simulink model "bu01_2018b"  (R2018b)
settings: Solver=VariableStepAuto  StartTime=0.0  StopTime=10.0  RelTol=1e-3
model workspace (MAT data in the model file):
  Ixx = 0.8
  Iyy = 2.075
  Izz = 1.25
  Mass = 11.5
libraries: aerolibutil x6, sharedtransform x4, simulink x3, sharedutil x3, shared6dof x1
(part 1 of 2)
settings Model: Creator=Administrator  LastModifiedBy=39926
settings DataIOCC: ReturnWorkspaceOutputs=on

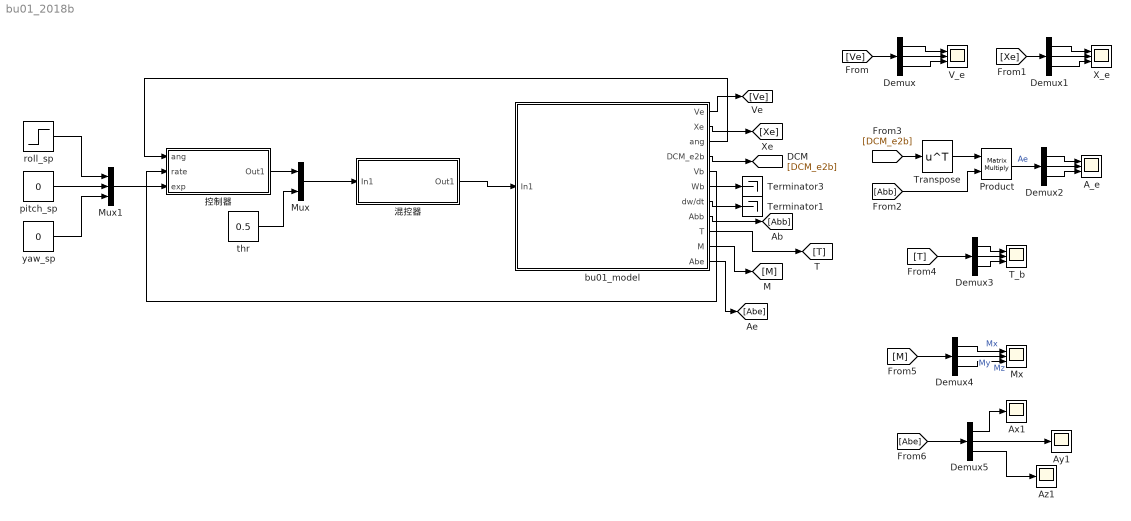
== system bu01_2018b ==
  A_e : Scope  NumInputPorts=3
  Ax1 : Scope
  Ay1 : Scope
  Az1 : Scope
  Demux{,1..5} (6 alike) : Demux  Outputs=3
  Mux : Mux  Inputs=2
  Mux1 : Mux  Inputs=3
  Mx : Scope  NumInputPorts=3
  Product : Product  Multiplication=Matrix(*)
  T_b : Scope  NumInputPorts=3
  Terminator1 : Terminator
  Terminator3 : Terminator
  Transpose : Math  Operator=transpose  SaturateOnIntegerOverflow=on
  V_e : Scope  NumInputPorts=3
  X_e : Scope  NumInputPorts=3
  bu01_model : Subsystem
  pitch_sp : Constant  Value=0
  roll_sp : Step  After=0  SampleTime=0
  thr : Constant  Value=0.5
  yaw_sp : Constant  Value=0
  控制器 : Subsystem
  混控器 : Subsystem
  wires:
  bu01_model/8(Abb) -> [Abb]
  bu01_model/7(dw/dt) -> Terminator1/1
  bu01_model/4(DCM_e2b) -> [DCM_e2b]
  bu01_model/5(Vb) -> Terminator3/1
  混控器/1(Out1) -> bu01_model/1(In1)
  Mux/1 -> 混控器/1(In1)
  bu01_model/3(ang) -> 控制器/1(ang)
  bu01_model/6(Wb) -> 控制器/2(rate)
  Mux1/1 -> 控制器/3(exp)
  控制器/1(Out1) -> Mux/1
  thr/1 -> Mux/2
  bu01_model/2(Xe) -> [Xe]
  Demux/1 -> V_e/1
  bu01_model/1(Ve) -> [Ve]
  [Ve] -> Demux/1
  [Xe] -> Demux1/1
  Demux1/1 -> X_e/1
  Demux1/2 -> X_e/2
  Demux1/3 -> X_e/3
  [DCM_e2b] -> Transpose/1
  Transpose/1 -> Product/1
  [Abb] -> Product/2
  Product/1 -> Demux2/1  "Ae"
  Demux2/1 -> A_e/1
  Demux2/2 -> A_e/2
  bu01_model/9(T) -> [T]
  bu01_model/10(M) -> [M]
  Demux3/3 -> T_b/3
  Demux3/2 -> T_b/2
  Demux3/1 -> T_b/1
  [T] -> Demux3/1
  [M] -> Demux4/1
  Demux4/1 -> Mx/1  "Mx"
  Demux4/2 -> Mx/2  "My"
  Demux4/3 -> Mx/3  "Mz"
  Demux2/3 -> A_e/3
  bu01_model/11(Abe) -> [Abe]
  Demux5/3 -> Az1/1
  Demux5/2 -> Ay1/1
  Demux5/1 -> Ax1/1
  [Abe] -> Demux5/1
  roll_sp/1 -> Mux1/1
  pitch_sp/1 -> Mux1/2
  yaw_sp/1 -> Mux1/3
  Demux/2 -> V_e/2
  Demux/3 -> V_e/3

== system bu01_2018b/bu01_model ==
  In1 : Inport
  6DOF (Quaternion) : shared6dof/6DOF (Euler Angles)  units=Metric (MKS)  mtype=Fixed  rep=Quaternion  xme_0=[0 0 0]  Vm_0=[0 0 0]  eul_0=[0 0 0]  pm_0=[0 0 0]  mass_0=Mass  mass_e=0.5  mass_f=2.0  inertia=[Ixx 0 0; 0 Iyy 0;0 0 Izz]  inertia_e=eye(3)  inertia_f=2*eye(3)  k_quat=1.0  vre_flag=on  abi_flag=on  aMode=0  xme_statename=''  Vm_statename=''  eul_statename=''  quat_statename=''  pm_statename=''  mass_statename=''
      settings: SourceProductBaseCode=AE
  力矩方程 : Subsystem
  推力方程 : Subsystem
  Ve : Outport
  Xe : Outport  Port=2
  ang : Outport  Port=3
  DCM_e2b : Outport  Port=4
  Vb : Outport  Port=5
  Wb : Outport  Port=6
  dw/dt : Outport  Port=7
  Abb : Outport  Port=8
  T : Outport  Port=9
  M : Outport  Port=10
  Abe : Outport  Port=11
  wires:
  力矩方程/1(Out1) -> M/1, 6DOF (Quaternion)/2
  6DOF (Quaternion)/1 -> Ve/1
  6DOF (Quaternion)/3 -> ang/1
  6DOF (Quaternion)/2 -> Xe/1
  6DOF (Quaternion)/4 -> 推力方程/2(DCM_e2b), DCM_e2b/1
  推力方程/1(Out1) -> T/1, 6DOF (Quaternion)/1
  6DOF (Quaternion)/7 -> dw/dt/1
  6DOF (Quaternion)/8 -> Abb/1
  6DOF (Quaternion)/5 -> Vb/1
  6DOF (Quaternion)/6 -> Wb/1
  In1/1 -> 推力方程/1(In1), 力矩方程/1(In1)
  6DOF (Quaternion)/9 -> Abe/1

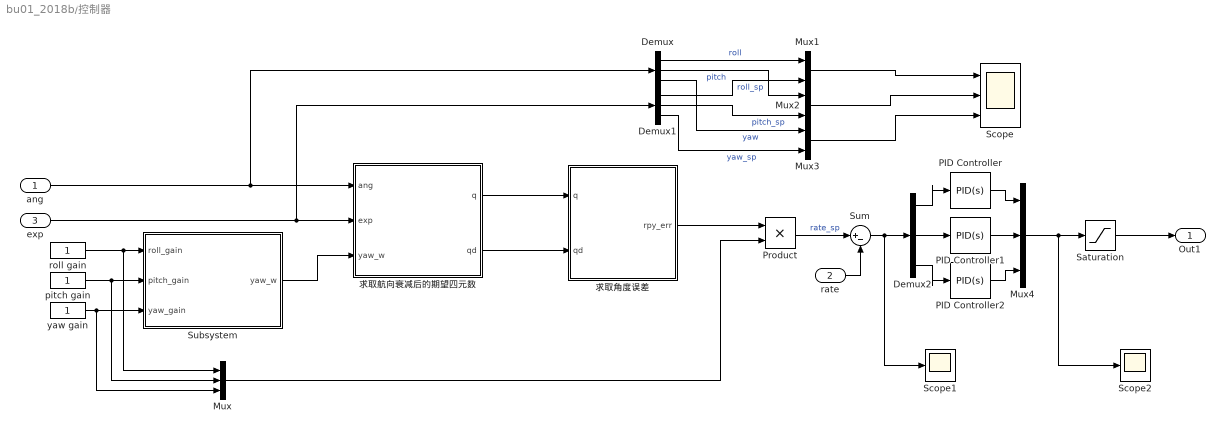
== system bu01_2018b/控制器 ==
  ang : Inport
  rate : Inport  Port=2
  exp : Inport  Port=3
  Demux : Demux  Outputs=3
  Demux1 : Demux  Outputs=3
  Demux2 : Demux  Outputs=3
  Mux : Mux  Inputs=3
  Mux1 : Mux  Inputs=2
  Mux2 : Mux  Inputs=2
  Mux3 : Mux  Inputs=2
  Mux4 : Mux  Inputs=3
  PID Controller : simulink/Continuous/PID Controller  Controller=PID  Form=Parallel  TimeDomain=Continuous-time  SampleTime=-1  IntegratorMethod=Forward Euler  FilterMethod=Forward Euler  ControllerParametersSource=internal  P=0.1  I=0.1  D=0  UseFilter=on  N=100  TunerSelectOption=Transfer Function Based (PID Tuner App)  InitialConditionSource=internal  InitialConditionForIntegrator=0  InitialConditionForFilter=0  DifferentiatorICPrevScaledInput=0  ExternalReset=none  TrackingMode=off  Kt=1  LimitOutput=off  UpperSaturationLimit=inf  LowerSaturationLimit=-inf  LinearizeAsGain=on  AntiWindupMode=none  Kb=1  POutMin=[]  POutMax=[]  IOutMin=[]  IOutMax=[]  DOutMin=[]  DOutMax=[]  NOutMin=[]  NOutMax=[]  SumOutMin=[]  SumOutMax=[]  SaturationOutMin=[]  SaturationOutMax=[]  PParamMin=[]  PParamMax=[]  IParamMin=[]  IParamMax=[]  DParamMin=[]  DParamMax=[]  NParamMin=[]  NParamMax=[]  KbParamMin=[]  KbParamMax=[]  KtParamMin=[]  KtParamMax=[]  KbOutMin=[]  KbOutMax=[]  KtOutMin=[]  KtOutMax=[]  IntegratorOutMin=[]  IntegratorOutMax=[]  FilterOutMin=[]  FilterOutMax=[]  SumI1OutMin=[]  SumI1OutMax=[]  SumI2OutMin=[]  SumI2OutMax=[]  SumI3OutMin=[]  SumI3OutMax=[]  SumI4OutMin=[]  SumI4OutMax=[]  SumDOutMin=[]  SumDOutMax=[]  DifferentiatorOutMin=[]  DifferentiatorOutMax=[]  FilterDiffOutCoefMin=[]  FilterDiffOutCoefMax=[]  ReciprocalOutMin=[]  ReciprocalOutMax=[]  SumDenOutMin=[]  SumDenOutMax=[]  SumNumOutMin=[]  SumNumOutMax=[]  DivideOutMin=[]  DivideOutMax=[]  IntegratorContinuousStateAttributes=''  IntegratorStateMustResolveToSignalObject=off  IntegratorRTWStateStorageClass=Auto  FilterContinuousStateAttributes=''  FilterStateMustResolveToSignalObject=off  FilterRTWStateStorageClass=Auto  ParallelPVariant=InternalParameters  IdealPVariant=Disabled  IVariant=InternalParameters  DVariant=InternalParameters  IntegratorVariant=Continuous  SatVariant=Disabled  AWVariant=Passthrough  PCopyVariant=Disabled  TRVariant=Disabled  FdbkBlocksVariant=Forward  IdealPFdbkVariant=Disabled  SatFdbkVariant=Disabled  DerivativeFilterVariant=ContFilter  NVariant=InternalParameters  NCopyVariant=Disabled  FilterICVariant=InternalICsFilter  IntegratorICVariant=InternalICs  ExternalResetVariant=Disabled  TRSumVariant=Passthrough  SumFdbkVariant=Disabled  SumVariant=Sum_PID
  PID Controller1 : simulink/Continuous/PID Controller  Controller=PID  Form=Parallel  TimeDomain=Continuous-time  SampleTime=-1  IntegratorMethod=Forward Euler  FilterMethod=Forward Euler  ControllerParametersSource=internal  P=0.15  I=0.1  D=0  UseFilter=on  N=100  TunerSelectOption=Transfer Function Based (PID Tuner App)  InitialConditionSource=internal  InitialConditionForIntegrator=0  InitialConditionForFilter=0  DifferentiatorICPrevScaledInput=0  ExternalReset=none  TrackingMode=off  Kt=1  LimitOutput=off  UpperSaturationLimit=inf  LowerSaturationLimit=-inf  LinearizeAsGain=on  AntiWindupMode=none  Kb=1  POutMin=[]  POutMax=[]  IOutMin=[]  IOutMax=[]  DOutMin=[]  DOutMax=[]  NOutMin=[]  NOutMax=[]  SumOutMin=[]  SumOutMax=[]  SaturationOutMin=[]  SaturationOutMax=[]  PParamMin=[]  PParamMax=[]  IParamMin=[]  IParamMax=[]  DParamMin=[]  DParamMax=[]  NParamMin=[]  NParamMax=[]  KbParamMin=[]  KbParamMax=[]  KtParamMin=[]  KtParamMax=[]  KbOutMin=[]  KbOutMax=[]  KtOutMin=[]  KtOutMax=[]  IntegratorOutMin=[]  IntegratorOutMax=[]  FilterOutMin=[]  FilterOutMax=[]  SumI1OutMin=[]  SumI1OutMax=[]  SumI2OutMin=[]  SumI2OutMax=[]  SumI3OutMin=[]  SumI3OutMax=[]  SumI4OutMin=[]  SumI4OutMax=[]  SumDOutMin=[]  SumDOutMax=[]  DifferentiatorOutMin=[]  DifferentiatorOutMax=[]  FilterDiffOutCoefMin=[]  FilterDiffOutCoefMax=[]  ReciprocalOutMin=[]  ReciprocalOutMax=[]  SumDenOutMin=[]  SumDenOutMax=[]  SumNumOutMin=[]  SumNumOutMax=[]  DivideOutMin=[]  DivideOutMax=[]  IntegratorContinuousStateAttributes=''  IntegratorStateMustResolveToSignalObject=off  IntegratorRTWStateStorageClass=Auto  FilterContinuousStateAttributes=''  FilterStateMustResolveToSignalObject=off  FilterRTWStateStorageClass=Auto  ParallelPVariant=InternalParameters  IdealPVariant=Disabled  IVariant=InternalParameters  DVariant=InternalParameters  IntegratorVariant=Continuous  SatVariant=Disabled  AWVariant=Passthrough  PCopyVariant=Disabled  TRVariant=Disabled  FdbkBlocksVariant=Forward  IdealPFdbkVariant=Disabled  SatFdbkVariant=Disabled  DerivativeFilterVariant=ContFilter  NVariant=InternalParameters  NCopyVariant=Disabled  FilterICVariant=InternalICsFilter  IntegratorICVariant=InternalICs  ExternalResetVariant=Disabled  TRSumVariant=Passthrough  SumFdbkVariant=Disabled  SumVariant=Sum_PID
  PID Controller2 : simulink/Continuous/PID Controller  Controller=PID  Form=Parallel  TimeDomain=Continuous-time  SampleTime=-1  IntegratorMethod=Forward Euler  FilterMethod=Forward Euler  ControllerParametersSource=internal  P=0.3  I=0.1  D=0  UseFilter=on  N=100  TunerSelectOption=Transfer Function Based (PID Tuner App)  InitialConditionSource=internal  InitialConditionForIntegrator=0  InitialConditionForFilter=0  DifferentiatorICPrevScaledInput=0  ExternalReset=none  TrackingMode=off  Kt=1  LimitOutput=off  UpperSaturationLimit=inf  LowerSaturationLimit=-inf  LinearizeAsGain=on  AntiWindupMode=none  Kb=1  POutMin=[]  POutMax=[]  IOutMin=[]  IOutMax=[]  DOutMin=[]  DOutMax=[]  NOutMin=[]  NOutMax=[]  SumOutMin=[]  SumOutMax=[]  SaturationOutMin=[]  SaturationOutMax=[]  PParamMin=[]  PParamMax=[]  IParamMin=[]  IParamMax=[]  DParamMin=[]  DParamMax=[]  NParamMin=[]  NParamMax=[]  KbParamMin=[]  KbParamMax=[]  KtParamMin=[]  KtParamMax=[]  KbOutMin=[]  KbOutMax=[]  KtOutMin=[]  KtOutMax=[]  IntegratorOutMin=[]  IntegratorOutMax=[]  FilterOutMin=[]  FilterOutMax=[]  SumI1OutMin=[]  SumI1OutMax=[]  SumI2OutMin=[]  SumI2OutMax=[]  SumI3OutMin=[]  SumI3OutMax=[]  SumI4OutMin=[]  SumI4OutMax=[]  SumDOutMin=[]  SumDOutMax=[]  DifferentiatorOutMin=[]  DifferentiatorOutMax=[]  FilterDiffOutCoefMin=[]  FilterDiffOutCoefMax=[]  ReciprocalOutMin=[]  ReciprocalOutMax=[]  SumDenOutMin=[]  SumDenOutMax=[]  SumNumOutMin=[]  SumNumOutMax=[]  DivideOutMin=[]  DivideOutMax=[]  IntegratorContinuousStateAttributes=''  IntegratorStateMustResolveToSignalObject=off  IntegratorRTWStateStorageClass=Auto  FilterContinuousStateAttributes=''  FilterStateMustResolveToSignalObject=off  FilterRTWStateStorageClass=Auto  ParallelPVariant=InternalParameters  IdealPVariant=Disabled  IVariant=InternalParameters  DVariant=InternalParameters  IntegratorVariant=Continuous  SatVariant=Disabled  AWVariant=Passthrough  PCopyVariant=Disabled  TRVariant=Disabled  FdbkBlocksVariant=Forward  IdealPFdbkVariant=Disabled  SatFdbkVariant=Disabled  DerivativeFilterVariant=ContFilter  NVariant=InternalParameters  NCopyVariant=Disabled  FilterICVariant=InternalICsFilter  IntegratorICVariant=InternalICs  ExternalResetVariant=Disabled  TRSumVariant=Passthrough  SumFdbkVariant=Disabled  SumVariant=Sum_PID
  Product : Product
  Saturation : Saturate  UpperLimit=1  LowerLimit=-1
  Scope : Scope  NumInputPorts=3
  Scope1 : Scope
  Scope2 : Scope
  Subsystem : Subsystem
  Sum : Sum  Inputs=|+-
  pitch gain : Constant
  roll gain : Constant
  yaw gain : Constant
  求取航向衰减后的期望四元数 : Subsystem
  求取角度误差 : Subsystem
  Out1 : Outport
  wires:
  ang/1 -> Demux/1, 求取航向衰减后的期望四元数/1(ang)
  exp/1 -> Demux1/1, 求取航向衰减后的期望四元数/2(exp)
  roll gain/1 -> Mux/1, Subsystem/1(roll_gain)
  pitch gain/1 -> Subsystem/2("pitch_gain "), Mux/2
  yaw gain/1 -> Subsystem/3(yaw_gain), Mux/3
  Subsystem/1(yaw_w) -> 求取航向衰减后的期望四元数/3("yaw_w ")
  求取航向衰减后的期望四元数/1(q) -> 求取角度误差/1(q)
  求取航向衰减后的期望四元数/2(qd) -> 求取角度误差/2(qd)
  求取角度误差/1(rpy_err) -> Product/1
  Mux/1 -> Product/2
  Product/1 -> Sum/1  "rate_sp"
  rate/1 -> Sum/2
  Sum/1 -> Scope1/1, Demux2/1
  Mux4/1 -> Scope2/1, Saturation/1
  Saturation/1 -> Out1/1
  Demux/1 -> Mux1/1  "roll"
  Demux1/1 -> Mux1/2  "roll_sp"
  Demux/2 -> Mux2/1  "pitch"
  Demux1/2 -> Mux2/2  "pitch_sp"
  Demux/3 -> Mux3/1  "yaw"
  Demux1/3 -> Mux3/2  "yaw_sp"
  Mux1/1 -> Scope/1
  Mux2/1 -> Scope/2
  Mux3/1 -> Scope/3
  Demux2/1 -> PID Controller/1
  Demux2/2 -> PID Controller1/1
  Demux2/3 -> PID Controller2/1
  PID Controller/1 -> Mux4/1
  PID Controller1/1 -> Mux4/2
  PID Controller2/1 -> Mux4/3

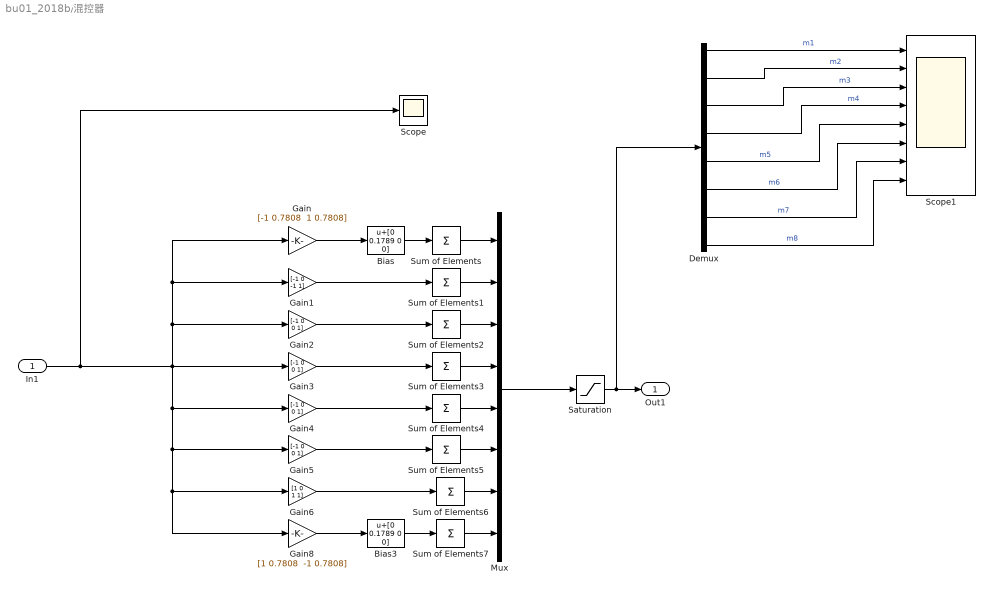
== system bu01_2018b/混控器 ==
  In1 : Inport
  Bias : Bias  Bias=[0 0.1789 0 0]
  Bias3 : Bias  Bias=[0 0.1789 0 0]
  Demux : Demux  Outputs=8
  Gain : Gain  Gain="[-1 0.7808  1 0.7808]"
  Gain1 : Gain  Gain="[-1 0  -1 1]"
  Gain{2..5} (4 alike) : Gain  Gain=[-1 0 0 1]
  Gain6 : Gain  Gain="[1 0  1 1]"
  Gain8 : Gain  Gain="[1 0.7808  -1 0.7808]"
  Mux : Mux  Inputs=8
  Saturation : Saturate  UpperLimit=1  LowerLimit=0
  Scope : Scope
  Scope1 : Scope  NumInputPorts=8
  Sum of Elements{,1..7} (8 alike) : Sum  Inputs=+
  Out1 : Outport
  wires:
  Sum of Elements/1 -> Mux/1
  Bias/1 -> Sum of Elements/1
  Gain2/1 -> Sum of Elements2/1
  Gain3/1 -> Sum of Elements3/1
  Gain5/1 -> Sum of Elements5/1
  Gain4/1 -> Sum of Elements4/1
  Mux/1 -> Saturation/1
  Gain/1 -> Bias/1
  Gain1/1 -> Sum of Elements1/1
  Gain6/1 -> Sum of Elements6/1
  Gain8/1 -> Bias3/1
  Bias3/1 -> Sum of Elements7/1
  Saturation/1 -> Demux/1, Out1/1
  Sum of Elements1/1 -> Mux/2
  Sum of Elements2/1 -> Mux/3
  Sum of Elements3/1 -> Mux/4
  Sum of Elements4/1 -> Mux/5
  Sum of Elements5/1 -> Mux/6
  Sum of Elements6/1 -> Mux/7
  Sum of Elements7/1 -> Mux/8
  In1/1 -> Scope/1, Gain3/1, Gain4/1, Gain5/1, Gain8/1, Gain6/1, Gain1/1, Gain/1, Gain2/1
  Demux/1 -> Scope1/1  "m1"
  Demux/2 -> Scope1/2  "m2"
  Demux/3 -> Scope1/3  "m3"
  Demux/4 -> Scope1/4  "m4"
  Demux/5 -> Scope1/5  "m5"
  Demux/6 -> Scope1/6  "m6"
  Demux/7 -> Scope1/7  "m7"
  Demux/8 -> Scope1/8  "m8"

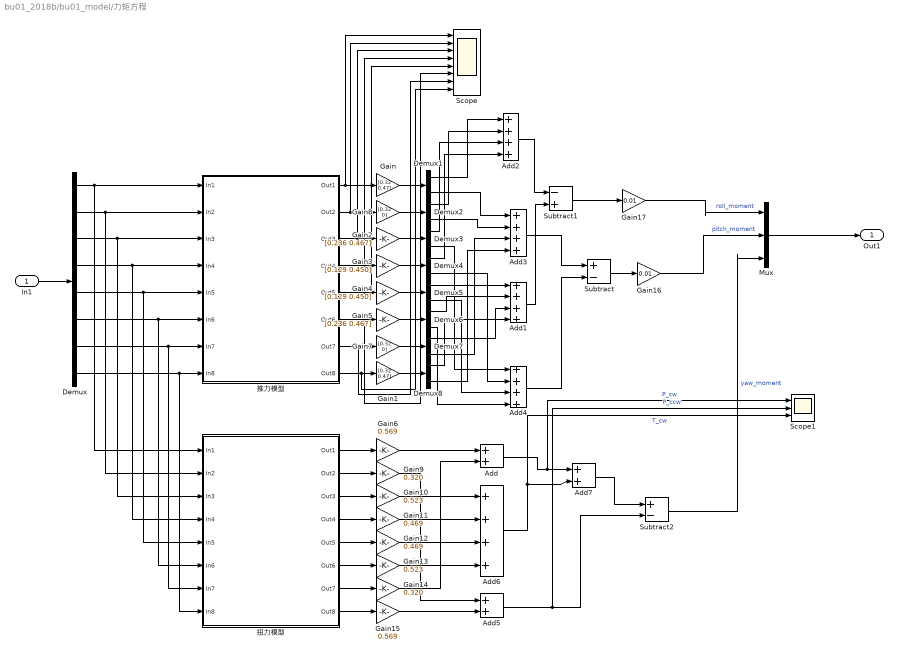
== system bu01_2018b/bu01_model/力矩方程 ==
  In1 : Inport
  Add : Sum
  Add{1..4} (4 alike) : Sum  Inputs=4
  Add5 : Sum
  Add6 : Sum  Inputs=++++
  Add7 : Sum
  Demux : Demux  Outputs=8
  Demux{1..8} (8 alike) : Demux  Outputs=2
  Gain : Gain  Gain=[0.32 0.47]
  Gain1 : Gain  Gain=[0.32 0.47]
  Gain10 : Gain  Gain=0.523
  Gain11 : Gain  Gain=0.469
  Gain12 : Gain  Gain=0.469
  Gain13 : Gain  Gain=0.523
  Gain14 : Gain  Gain=0.320
  Gain15 : Gain  Gain=0.569
  Gain16 : Gain  Gain=0.01
  Gain17 : Gain  Gain=0.01
  Gain2 : Gain  Gain=[0.236 0.467]
  Gain3 : Gain  Gain=[0.129 0.450]
  Gain4 : Gain  Gain=[0.129 0.450]
  Gain5 : Gain  Gain=[0.236 0.467]
  Gain6 : Gain  Gain=0.569
  Gain7 : Gain  Gain=[0.32 0]
  Gain8 : Gain  Gain=[0.32 0]
  Gain9 : Gain  Gain=0.320
  Mux : Mux  Inputs=3
  Scope : Scope  NumInputPorts=8
  Scope1 : Scope  NumInputPorts=3
  Subtract : Sum  Inputs=+-
  Subtract1 : Sum  Inputs=-+
  Subtract2 : Sum  Inputs=+-
  扭力模型 : Subsystem
  推力模型 : Subsystem
  Out1 : Outport
  wires:
  In1/1 -> Demux/1
  Demux/1 -> 推力模型/1(In1), 扭力模型/1(In1)
  Demux/2 -> 扭力模型/2(In2), 推力模型/2(In2)
  Demux/3 -> 推力模型/3(In3), 扭力模型/3(In3)
  Demux/4 -> 推力模型/4(In4), 扭力模型/4(In4)
  Demux/5 -> 推力模型/5(In5), 扭力模型/5(In5)
  Demux/6 -> 扭力模型/6(In6), 推力模型/6(In6)
  Demux/7 -> 扭力模型/7(In7), 推力模型/7(In7)
  Demux/8 -> 扭力模型/8(In8), 推力模型/8(In8)
  推力模型/1(Out1) -> Scope/1, Gain/1
  推力模型/8(Out8) -> Scope/8, Gain1/1
  推力模型/4(Out4) -> Scope/4, Gain3/1
  推力模型/5(Out5) -> Scope/5, Gain4/1
  推力模型/6(Out6) -> Scope/6, Gain5/1
  推力模型/7(Out7) -> Scope/7, Gain7/1
  Gain/1 -> Demux1/1
  Gain8/1 -> Demux2/1
  Gain2/1 -> Demux3/1
  Gain3/1 -> Demux4/1
  Gain4/1 -> Demux5/1
  Gain5/1 -> Demux6/1
  Gain7/1 -> Demux7/1
  Gain1/1 -> Demux8/1
  Demux1/1 -> Add2/1
  Demux2/1 -> Add2/2
  Demux3/1 -> Add2/3
  Demux4/1 -> Add2/4
  Demux5/1 -> Add1/1
  Demux6/1 -> Add1/2
  Demux7/1 -> Add1/3
  Demux8/1 -> Add1/4
  Add2/1 -> Subtract1/1
  Add1/1 -> Subtract1/2
  Demux1/2 -> Add3/1
  Demux2/2 -> Add3/2
  Demux7/2 -> Add3/3
  Demux8/2 -> Add3/4
  Demux3/2 -> Add4/1
  Demux4/2 -> Add4/2
  Demux5/2 -> Add4/3
  Demux6/2 -> Add4/4
  Add3/1 -> Subtract/1
  Add4/1 -> Subtract/2
  扭力模型/1(Out1) -> Gain6/1
  扭力模型/2(Out2) -> Gain9/1
  扭力模型/3(Out3) -> Gain10/1
  扭力模型/4(Out4) -> Gain11/1
  扭力模型/5(Out5) -> Gain12/1
  扭力模型/6(Out6) -> Gain13/1
  扭力模型/7(Out7) -> Gain14/1
  扭力模型/8(Out8) -> Gain15/1
  Gain6/1 -> Add/1
  Gain14/1 -> Add/2
  Gain15/1 -> Add5/2
  Gain9/1 -> Add5/1
  Gain13/1 -> Add6/4
  Gain12/1 -> Add6/3
  Gain11/1 -> Add6/2
  Gain10/1 -> Add6/1
  Add/1 -> Scope1/1, Add7/1  "P_cw"
  Add7/1 -> Subtract2/1
  Add5/1 -> Scope1/2, Subtract2/2  "P_ccw"
  Subtract2/1 -> Mux/3  "yaw_moment"
  Mux/1 -> Out1/1
  Subtract/1 -> Gain16/1
  Gain16/1 -> Mux/2  "pitch_moment"
  Subtract1/1 -> Gain17/1
  Gain17/1 -> Mux/1  "roll_moment"
  推力模型/2(Out2) -> Gain8/1, Scope/2
  推力模型/3(Out3) -> Scope/3, Gain2/1
  Add6/1 -> Scope1/3, Add7/2  "T_cw"

== system bu01_2018b/bu01_model/推力方程 ==
  In1 : Inport
  DCM_e2b : Inport  Port=2
  Add : Sum  Inputs=8
  Add1 : Sum
  Constant : Constant  Value=0
  Constant1 : Constant  Value=0
  Demux : Demux  Outputs=8
  Gain : Gain  Gain=-0.01
  Mux : Mux  Inputs=3
  Product : Product  Multiplication=Matrix(*)
  aircraft_mg : Constant  Value=[0 0 115.7]
  动力模型 : Subsystem
  Out1 : Outport
  wires:
  In1/1 -> Demux/1
  Demux/1 -> 动力模型/1(In1)
  Demux/2 -> 动力模型/2(In2)
  Demux/3 -> 动力模型/3(In3)
  Demux/4 -> 动力模型/4(In4)
  Demux/5 -> 动力模型/5(In5)
  Demux/6 -> 动力模型/6(In6)
  Demux/7 -> 动力模型/7(In7)
  Demux/8 -> 动力模型/8(In8)
  动力模型/1(Out1) -> Add/1
  动力模型/2(Out2) -> Add/2
  动力模型/3(Out3) -> Add/3
  动力模型/4(Out4) -> Add/4
  动力模型/5(Out5) -> Add/5
  动力模型/7(Out7) -> Add/7
  动力模型/6(Out6) -> Add/6
  动力模型/8(Out8) -> Add/8
  Constant/1 -> Mux/1
  Constant1/1 -> Mux/2
  Add/1 -> Gain/1
  Gain/1 -> Mux/3
  DCM_e2b/1 -> Product/1
  aircraft_mg/1 -> Product/2
  Product/1 -> Add1/2
  Mux/1 -> Add1/1
  Add1/1 -> Out1/1

== system bu01_2018b/控制器/Subsystem ==
  note: 将比例增益当做系统时间常数，用其比例关系作为控制器衰减比例
  roll_gain : Inport
  "pitch_gain " : Inport  Port=2
  yaw_gain : Inport  Port=3
  Add : Sum
  Divide : Product  Inputs=*/
  Gain : Gain  Gain=0.5
  Saturation : Saturate  UpperLimit=1  LowerLimit=0
  yaw_w : Outport
  wires:
  roll_gain/1 -> Add/1
  Add/1 -> Gain/1
  "pitch_gain "/1 -> Add/2
  Gain/1 -> Divide/2
  yaw_gain/1 -> Divide/1
  Divide/1 -> Saturation/1
  Saturation/1 -> yaw_w/1

== system bu01_2018b/控制器/求取航向衰减后的期望四元数 ==
  ang : Inport
  exp : Inport  Port=2
  "yaw_w " : Inport  Port=3
  MATLAB Function : MATLAB Function  TreatAsAtomicUnit=on
  Quaternion Normalize : sharedutil/Quaternion Normalize  aMode=aMode
      settings: SourceProductName=Aerospace Blockset  SourceProductBaseCode=AE
  求取只要倾斜的运动的期望四元数 : Subsystem
  求取绕机体Z轴旋转的误差四元数 : Subsystem
  获取地球系下当前机体系Z轴矢量 : Subsystem
  获取地球系下期望机体系Z轴矢量 : Subsystem
  计算航向衰减后的期望四元数 : Subsystem
  q : Outport
  qd : Outport  Port=2
  wires:
  获取地球系下当前机体系Z轴矢量/2(e_z) -> MATLAB Function/1(src)
  ang/1 -> 获取地球系下当前机体系Z轴矢量/1(ang)
  exp/1 -> 获取地球系下期望机体系Z轴矢量/1(exp)
  获取地球系下当前机体系Z轴矢量/1(q) -> q/1, 求取只要倾斜的运动的期望四元数/1(q)
  获取地球系下期望机体系Z轴矢量/1(e_z_d) -> MATLAB Function/2(dst)
  获取地球系下期望机体系Z轴矢量/2("qd ") -> 求取绕机体Z轴旋转的误差四元数/2(qd), 求取只要倾斜的运动的期望四元数/3(qd)
  "yaw_w "/1 -> 计算航向衰减后的期望四元数/1(yaw_w)
  求取绕机体Z轴旋转的误差四元数/1(q_mix_sign) -> 计算航向衰减后的期望四元数/3(q_mix_sign)
  计算航向衰减后的期望四元数/1(qd) -> qd/1
  求取只要倾斜的运动的期望四元数/1(qd_red_update) -> 计算航向衰减后的期望四元数/2(q_red_update), 求取绕机体Z轴旋转的误差四元数/1(qd_red_update)
  MATLAB Function/1(q) -> Quaternion Normalize/1  "qd_red"
  Quaternion Normalize/1 -> 求取只要倾斜的运动的期望四元数/2(qd_red)

== system bu01_2018b/控制器/求取角度误差 ==
  q : Inport
  qd : Inport  Port=2
  Constant : Constant  Value=0
  Gain : Gain  Gain=-1
  Gain1 : Gain  Gain=2
  GreaterThanOrEqual : RelationalOperator  OutDataTypeStr=boolean  RndMeth=Simplest
  Quaternion Inverse : aerolibutil/Quaternion Inverse
      settings: SourceProductName=Aerospace Blockset
  Quaternion Multiplication : aerolibutil/Quaternion Multiplication
  Selector : Selector  InputPortWidth=4  IndexOptions=Index vector (dialog)  Indices=1  OutputSizes=1
  Selector1 : Selector  InputPortWidth=4  IndexOptions=Index vector (dialog)  Indices=[2 3 4]  OutputSizes=1
  Switch : Switch  Criteria=u2 > Threshold
  rpy_err : Outport
  wires:
  Quaternion Inverse/1 -> Quaternion Multiplication/1
  q/1 -> Quaternion Inverse/1
  Quaternion Multiplication/1 -> Selector1/1, Selector/1  "quat_err"
  qd/1 -> Quaternion Multiplication/2
  Selector/1 -> GreaterThanOrEqual/1
  Constant/1 -> GreaterThanOrEqual/2
  GreaterThanOrEqual/1 -> Switch/2
  Selector1/1 -> Switch/1, Gain/1
  Gain/1 -> Switch/3
  Switch/1 -> Gain1/1
  Gain1/1 -> rpy_err/1  "ang_err"

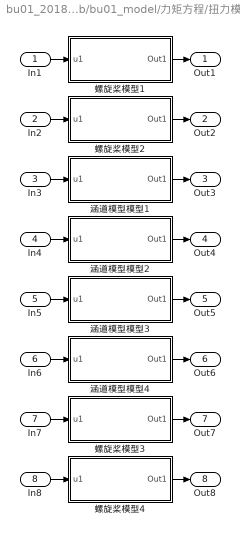
== system bu01_2018b/bu01_model/力矩方程/扭力模型 ==
  In1 : Inport
  In2 : Inport  Port=2
  In3 : Inport  Port=3
  In4 : Inport  Port=4
  In5 : Inport  Port=5
  In6 : Inport  Port=6
  In7 : Inport  Port=7
  In8 : Inport  Port=8
  涵道模型模型1 : Subsystem
  涵道模型模型2 : Subsystem
  涵道模型模型3 : Subsystem
  涵道模型模型4 : Subsystem
  螺旋桨模型1 : Subsystem
  螺旋桨模型2 : Subsystem
  螺旋桨模型3 : Subsystem
  螺旋桨模型4 : Subsystem
  Out1 : Outport
  Out2 : Outport  Port=2
  Out3 : Outport  Port=3
  Out4 : Outport  Port=4
  Out5 : Outport  Port=5
  Out6 : Outport  Port=6
  Out7 : Outport  Port=7
  Out8 : Outport  Port=8
  wires:
  In3/1 -> 涵道模型模型1/1(u1)
  涵道模型模型2/1(Out1) -> Out4/1
  涵道模型模型3/1(Out1) -> Out5/1
  螺旋桨模型1/1(Out1) -> Out1/1
  In7/1 -> 螺旋桨模型3/1(u1)
  涵道模型模型1/1(Out1) -> Out3/1
  In4/1 -> 涵道模型模型2/1(u1)
  In5/1 -> 涵道模型模型3/1(u1)
  螺旋桨模型3/1(Out1) -> Out7/1
  In2/1 -> 螺旋桨模型2/1(u1)
  螺旋桨模型2/1(Out1) -> Out2/1
  In6/1 -> 涵道模型模型4/1(u1)
  涵道模型模型4/1(Out1) -> Out6/1
  螺旋桨模型4/1(Out1) -> Out8/1
  In8/1 -> 螺旋桨模型4/1(u1)
  In1/1 -> 螺旋桨模型1/1(u1)

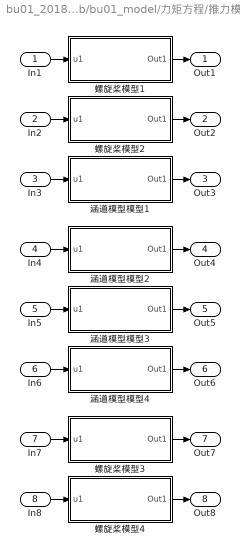
== system bu01_2018b/bu01_model/力矩方程/推力模型 ==
  In1 : Inport
  In2 : Inport  Port=2
  In3 : Inport  Port=3
  In4 : Inport  Port=4
  In5 : Inport  Port=5
  In6 : Inport  Port=6
  In7 : Inport  Port=7
  In8 : Inport  Port=8
  涵道模型模型1 : Subsystem
  涵道模型模型2 : Subsystem
  涵道模型模型3 : Subsystem
  涵道模型模型4 : Subsystem
  螺旋桨模型1 : Subsystem
  螺旋桨模型2 : Subsystem
  螺旋桨模型3 : Subsystem
  螺旋桨模型4 : Subsystem
  Out1 : Outport
  Out2 : Outport  Port=2
  Out3 : Outport  Port=3
  Out4 : Outport  Port=4
  Out5 : Outport  Port=5
  Out6 : Outport  Port=6
  Out7 : Outport  Port=7
  Out8 : Outport  Port=8
  wires:
  In2/1 -> 螺旋桨模型2/1(u1)
  In3/1 -> 涵道模型模型1/1(u1)
  In7/1 -> 螺旋桨模型3/1(u1)
  In1/1 -> 螺旋桨模型1/1(u1)
  螺旋桨模型1/1(Out1) -> Out1/1
  涵道模型模型1/1(Out1) -> Out3/1
  In8/1 -> 螺旋桨模型4/1(u1)
  涵道模型模型3/1(Out1) -> Out5/1
  螺旋桨模型4/1(Out1) -> Out8/1
  In6/1 -> 涵道模型模型4/1(u1)
  螺旋桨模型3/1(Out1) -> Out7/1
  螺旋桨模型2/1(Out1) -> Out2/1
  In5/1 -> 涵道模型模型3/1(u1)
  涵道模型模型4/1(Out1) -> Out6/1
  涵道模型模型2/1(Out1) -> Out4/1
  In4/1 -> 涵道模型模型2/1(u1)

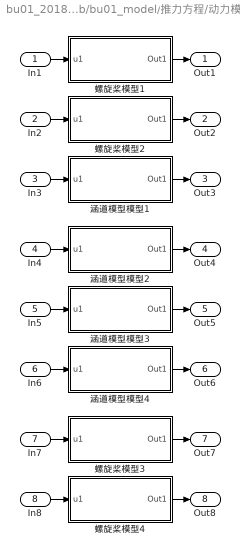
== system bu01_2018b/bu01_model/推力方程/动力模型 ==
  In1 : Inport
  In2 : Inport  Port=2
  In3 : Inport  Port=3
  In4 : Inport  Port=4
  In5 : Inport  Port=5
  In6 : Inport  Port=6
  In7 : Inport  Port=7
  In8 : Inport  Port=8
  涵道模型模型1 : Subsystem
  涵道模型模型2 : Subsystem
  涵道模型模型3 : Subsystem
  涵道模型模型4 : Subsystem
  螺旋桨模型1 : Subsystem
  螺旋桨模型2 : Subsystem
  螺旋桨模型3 : Subsystem
  螺旋桨模型4 : Subsystem
  Out1 : Outport
  Out2 : Outport  Port=2
  Out3 : Outport  Port=3
  Out4 : Outport  Port=4
  Out5 : Outport  Port=5
  Out6 : Outport  Port=6
  Out7 : Outport  Port=7
  Out8 : Outport  Port=8
  wires:
  In2/1 -> 螺旋桨模型2/1(u1)
  In3/1 -> 涵道模型模型1/1(u1)
  In7/1 -> 螺旋桨模型3/1(u1)
  In1/1 -> 螺旋桨模型1/1(u1)
  螺旋桨模型1/1(Out1) -> Out1/1
  涵道模型模型1/1(Out1) -> Out3/1
  In8/1 -> 螺旋桨模型4/1(u1)
  涵道模型模型3/1(Out1) -> Out5/1
  螺旋桨模型4/1(Out1) -> Out8/1
  In6/1 -> 涵道模型模型4/1(u1)
  螺旋桨模型3/1(Out1) -> Out7/1
  螺旋桨模型2/1(Out1) -> Out2/1
  In5/1 -> 涵道模型模型3/1(u1)
  涵道模型模型4/1(Out1) -> Out6/1
  涵道模型模型2/1(Out1) -> Out4/1
  In4/1 -> 涵道模型模型2/1(u1)

== system bu01_2018b/控制器/求取航向衰减后的期望四元数/求取只要倾斜的运动的期望四元数 ==
  note: 没有航向旋转的情况
  q : Inport
  qd_red : Inport  Port=2
  qd : Inport  Port=3
  Constant : Constant  Value=1-1e-5
  Demux : Demux  Outputs=2
  GreaterThan : RelationalOperator  Operator=>  OutDataTypeStr=boolean  RndMeth=Simplest
  GreaterThan1 : RelationalOperator  Operator=>  OutDataTypeStr=boolean  RndMeth=Simplest
  OR : Logic  Operator=OR  IconShape=distinctive  AllPortsSameDT=off  OutDataTypeStr=boolean
  Quaternion Multiplication : aerolibutil/Quaternion Multiplication
  Selector : Selector  InputPortWidth=4  IndexOptions=Index vector (dialog)  Indices=[2 3]  OutputSizes=1
  Switch : Switch  Criteria=u2 > Threshold
  qd_red_update : Outport
  wires:
  qd/1 -> Switch/1
  Constant/1 -> GreaterThan/2, GreaterThan1/2
  GreaterThan/1 -> OR/1
  q/1 -> Quaternion Multiplication/2
  GreaterThan1/1 -> OR/2
  qd_red/1 -> Quaternion Multiplication/1, Selector/1
  OR/1 -> Switch/2
  Demux/2 -> GreaterThan1/1
  Demux/1 -> GreaterThan/1
  Selector/1 -> Demux/1
  Quaternion Multiplication/1 -> Switch/3
  Switch/1 -> qd_red_update/1  "qd_red_update"

== system bu01_2018b/控制器/求取航向衰减后的期望四元数/求取绕机体Z轴旋转的误差四元数 ==
  qd_red_update : Inport
  qd : Inport  Port=2
  Constant1 : Constant  Value=0
  Gain : Gain  Gain=-1
  GreaterThan2 : RelationalOperator  OutDataTypeStr=boolean  RndMeth=Simplest
  Quaternion Inverse : aerolibutil/Quaternion Inverse
      settings: SourceProductName=Aerospace Blockset
  Quaternion Multiplication1 : aerolibutil/Quaternion Multiplication
  Selector1 : Selector  InputPortWidth=4  IndexOptions=Index vector (dialog)  Indices=1  OutputSizes=1
  Switch1 : Switch  Criteria=u2 > Threshold
  q_mix_sign : Outport
  wires:
  qd/1 -> Quaternion Multiplication1/2
  Quaternion Multiplication1/1 -> Gain/1, Switch1/1, Selector1/1  "q_mix"
  Gain/1 -> Switch1/3
  Selector1/1 -> GreaterThan2/1
  GreaterThan2/1 -> Switch1/2
  Constant1/1 -> GreaterThan2/2
  Quaternion Inverse/1 -> Quaternion Multiplication1/1
  qd_red_update/1 -> Quaternion Inverse/1
  Switch1/1 -> q_mix_sign/1  "q_mix_sign"

== system bu01_2018b/控制器/求取航向衰减后的期望四元数/获取地球系下当前机体系Z轴矢量 ==
  ang : Inport
  Quaternion Normalize1 : sharedutil/Quaternion Normalize  aMode=aMode
      settings: SourceProductName=Aerospace Blockset  SourceProductBaseCode=AE
  Quaternions to Direction Cosine Matrix1 : sharedtransform/Quaternions to  Direction Cosine Matrix  aMode=aMode
      settings: SourceProductName=Aerospace Blockset  SourceProductBaseCode=AE
  Rotation Angles to Quaternions : sharedtransform/Rotation Angles to Quaternions  rotationOrder=XYZ  aMode=aMode
      settings: SourceProductName=Aerospace Blockset  SourceProductBaseCode=AE
  提取机体系Z轴在 导航系下的矢量1 : Selector  NumberOfDimensions=2  InputPortWidth=3  IndexOptions=Index vector (dialog),Index vector (dialog)  Indices=3,[1 2 3]  OutputSizes=1,1
  q : Outport
  e_z : Outport  Port=2
  wires:
  Quaternions to Direction Cosine Matrix1/1 -> 提取机体系Z轴在 导航系下的矢量1/1
  Quaternion Normalize1/1 -> q/1, Quaternions to Direction Cosine Matrix1/1
  Rotation Angles to Quaternions/1 -> Quaternion Normalize1/1
  ang/1 -> Rotation Angles to Quaternions/1
  提取机体系Z轴在 导航系下的矢量1/1 -> e_z/1

== system bu01_2018b/控制器/求取航向衰减后的期望四元数/获取地球系下期望机体系Z轴矢量 ==
  exp : Inport
  Quaternion Normalize : sharedutil/Quaternion Normalize  aMode=aMode
      settings: SourceProductName=Aerospace Blockset  SourceProductBaseCode=AE
  Quaternions to Direction Cosine Matrix : sharedtransform/Quaternions to  Direction Cosine Matrix  aMode=aMode
      settings: SourceProductName=Aerospace Blockset  SourceProductBaseCode=AE
  Rotation Angles to Quaternions1 : sharedtransform/Rotation Angles to Quaternions  rotationOrder=XYZ  aMode=aMode
      settings: SourceProductName=Aerospace Blockset  SourceProductBaseCode=AE
  提取机体系Z轴在 导航系下的矢量 : Selector  NumberOfDimensions=2  InputPortWidth=3  IndexOptions=Index vector (dialog),Index vector (dialog)  Indices=3,[1 2 3]  OutputSizes=1,1
  e_z_d : Outport
  "qd " : Outport  Port=2
  wires:
  Rotation Angles to Quaternions1/1 -> Quaternion Normalize/1
  Quaternion Normalize/1 -> "qd "/1, Quaternions to Direction Cosine Matrix/1
  Quaternions to Direction Cosine Matrix/1 -> 提取机体系Z轴在 导航系下的矢量/1
  提取机体系Z轴在 导航系下的矢量/1 -> e_z_d/1
  exp/1 -> Rotation Angles to Quaternions1/1

== system bu01_2018b/控制器/求取航向衰减后的期望四元数/计算航向衰减后的期望四元数 ==
  yaw_w : Inport
  q_red_update : Inport  Port=2
  q_mix_sign : Inport  Port=3
  Acos : Trigonometry  Operator=acos
  Acos1 : Trigonometry  Operator=asin
  Constant3 : Constant  Value=0
  Cos : Trigonometry  Operator=cos
  Cos1 : Trigonometry
  Demux1 : Demux  Outputs=2
  Mux : Mux
  Product : Product
  Product1 : Product
  Quaternion Multiplication2 : aerolibutil/Quaternion Multiplication
  Saturation : Saturate  UpperLimit=1  LowerLimit=-1
  Selector2 : Selector  InputPortWidth=4  IndexOptions=Index vector (dialog)  Indices=[1 4]  OutputSizes=1
  qd : Outport
  wires:
  Product/1 -> Cos/1
  Cos/1 -> Mux/1
  Cos1/1 -> Mux/4
  Saturation/1 -> Demux1/1
  yaw_w/1 -> Product1/2, Product/1
  Acos/1 -> Product/2
  Demux1/1 -> Acos/1
  Product1/1 -> Cos1/1
  Mux/1 -> Quaternion Multiplication2/2
  Quaternion Multiplication2/1 -> qd/1  "qd"
  Constant3/1 -> Mux/3, Mux/2
  Acos1/1 -> Product1/1
  q_red_update/1 -> Quaternion Multiplication2/1
  Demux1/2 -> Acos1/1
  Selector2/1 -> Saturation/1
  q_mix_sign/1 -> Selector2/1

== system bu01_2018b/bu01_model/力矩方程/扭力模型/涵道模型模型1 ==
  u1 : Inport
  Add : Sum
  Constant : Constant  Value=0
  Constant1 : Constant  Value=0.1023
  Constant2 : Constant  Value=0.1023
  Constant3 : Constant
  Gain : Gain  Gain=0.003
  Gain1 : Gain  Gain=0.09767
  Gain2 : Gain  Gain=20
  MATLAB Function : MATLAB Function  TreatAsAtomicUnit=on
  MATLAB Function1 : MATLAB Function  TreatAsAtomicUnit=on
  Out1 : Outport
  wires:
  MATLAB Function1/1(y) -> Gain1/1
  Constant2/1 -> MATLAB Function1/2(a)
  Constant3/1 -> MATLAB Function1/3(b)
  Constant1/1 -> MATLAB Function/3(b)
  Gain1/1 -> Add/2
  Constant/1 -> MATLAB Function/2(a)
  u1/1 -> MATLAB Function1/1(u), MATLAB Function/1(u)
  Gain/1 -> Add/1
  MATLAB Function/1(y) -> Gain/1
  Add/1 -> Gain2/1
  Gain2/1 -> Out1/1

== system bu01_2018b/bu01_model/力矩方程/扭力模型/涵道模型模型2 ==
  u1 : Inport
  Add : Sum
  Constant : Constant  Value=0
  Constant1 : Constant  Value=0.1023
  Constant2 : Constant  Value=0.1023
  Constant3 : Constant
  Gain : Gain  Gain=0.003
  Gain1 : Gain  Gain=0.09767
  Gain2 : Gain  Gain=20
  MATLAB Function : MATLAB Function  TreatAsAtomicUnit=on
  MATLAB Function1 : MATLAB Function  TreatAsAtomicUnit=on
  Out1 : Outport
  wires:
  Gain2/1 -> Out1/1
  Add/1 -> Gain2/1
  MATLAB Function/1(y) -> Gain/1
  Gain/1 -> Add/1
  u1/1 -> MATLAB Function/1(u), MATLAB Function1/1(u)
  Constant/1 -> MATLAB Function/2(a)
  Gain1/1 -> Add/2
  Constant1/1 -> MATLAB Function/3(b)
  Constant3/1 -> MATLAB Function1/3(b)
  Constant2/1 -> MATLAB Function1/2(a)
  MATLAB Function1/1(y) -> Gain1/1

== system bu01_2018b/bu01_model/力矩方程/扭力模型/涵道模型模型3 ==
  u1 : Inport
  Add : Sum
  Constant : Constant  Value=0
  Constant1 : Constant  Value=0.1023
  Constant2 : Constant  Value=0.1023
  Constant3 : Constant
  Gain : Gain  Gain=0.003
  Gain1 : Gain  Gain=0.09767
  Gain2 : Gain  Gain=20
  MATLAB Function : MATLAB Function  TreatAsAtomicUnit=on
  MATLAB Function1 : MATLAB Function  TreatAsAtomicUnit=on
  Out1 : Outport
  wires:
  MATLAB Function1/1(y) -> Gain1/1
  Constant2/1 -> MATLAB Function1/2(a)
  Constant3/1 -> MATLAB Function1/3(b)
  Constant1/1 -> MATLAB Function/3(b)
  Gain1/1 -> Add/2
  Constant/1 -> MATLAB Function/2(a)
  u1/1 -> MATLAB Function1/1(u), MATLAB Function/1(u)
  Gain/1 -> Add/1
  MATLAB Function/1(y) -> Gain/1
  Add/1 -> Gain2/1
  Gain2/1 -> Out1/1

== system bu01_2018b/bu01_model/力矩方程/扭力模型/涵道模型模型4 ==
  u1 : Inport
  Add : Sum
  Constant : Constant  Value=0
  Constant1 : Constant  Value=0.1023
  Constant2 : Constant  Value=0.1023
  Constant3 : Constant
  Gain : Gain  Gain=0.003
  Gain1 : Gain  Gain=0.09767
  Gain2 : Gain  Gain=20
  MATLAB Function : MATLAB Function  TreatAsAtomicUnit=on
  MATLAB Function1 : MATLAB Function  TreatAsAtomicUnit=on
  Out1 : Outport
  wires:
  Gain2/1 -> Out1/1
  Add/1 -> Gain2/1
  MATLAB Function/1(y) -> Gain/1
  Gain/1 -> Add/1
  u1/1 -> MATLAB Function/1(u), MATLAB Function1/1(u)
  Constant/1 -> MATLAB Function/2(a)
  Gain1/1 -> Add/2
  Constant1/1 -> MATLAB Function/3(b)
  Constant3/1 -> MATLAB Function1/3(b)
  Constant2/1 -> MATLAB Function1/2(a)
  MATLAB Function1/1(y) -> Gain1/1

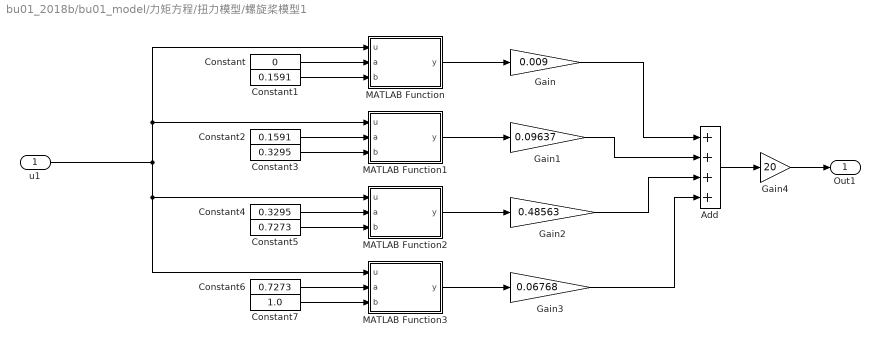
== system bu01_2018b/bu01_model/力矩方程/扭力模型/螺旋桨模型1 ==
  u1 : Inport
  Add : Sum  Inputs=4
  Constant : Constant  Value=0
  Constant1 : Constant  Value=0.1591
  Constant2 : Constant  Value=0.1591
  Constant3 : Constant  Value=0.3295
  Constant4 : Constant  Value=0.3295
  Constant5 : Constant  Value=0.7273
  Constant6 : Constant  Value=0.7273
  Constant7 : Constant  Value=1.0
  Gain : Gain  Gain=0.009
  Gain1 : Gain  Gain=0.09637
  Gain2 : Gain  Gain=0.48563
  Gain3 : Gain  Gain=0.06768
  Gain4 : Gain  Gain=20
  MATLAB Function : MATLAB Function  TreatAsAtomicUnit=on
  MATLAB Function1 : MATLAB Function  TreatAsAtomicUnit=on
  MATLAB Function2 : MATLAB Function  TreatAsAtomicUnit=on
  MATLAB Function3 : MATLAB Function  TreatAsAtomicUnit=on
  Out1 : Outport
  wires:
  u1/1 -> MATLAB Function1/1(u), MATLAB Function/1(u), MATLAB Function2/1(u), MATLAB Function3/1(u)
  Gain3/1 -> Add/4
  Gain2/1 -> Add/3
  Gain1/1 -> Add/2
  Gain/1 -> Add/1
  Constant7/1 -> MATLAB Function3/3(b)
  Constant6/1 -> MATLAB Function3/2(a)
  Constant5/1 -> MATLAB Function2/3(b)
  Constant4/1 -> MATLAB Function2/2(a)
  Constant3/1 -> MATLAB Function1/3(b)
  Constant2/1 -> MATLAB Function1/2(a)
  Constant1/1 -> MATLAB Function/3(b)
  Constant/1 -> MATLAB Function/2(a)
  MATLAB Function3/1(y) -> Gain3/1
  MATLAB Function2/1(y) -> Gain2/1
  MATLAB Function1/1(y) -> Gain1/1
  MATLAB Function/1(y) -> Gain/1
  Add/1 -> Gain4/1
  Gain4/1 -> Out1/1

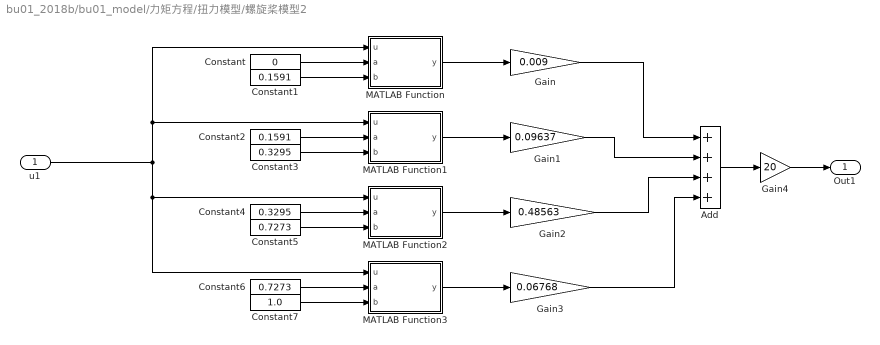
== system bu01_2018b/bu01_model/力矩方程/扭力模型/螺旋桨模型2 ==
  u1 : Inport
  Add : Sum  Inputs=4
  Constant : Constant  Value=0
  Constant1 : Constant  Value=0.1591
  Constant2 : Constant  Value=0.1591
  Constant3 : Constant  Value=0.3295
  Constant4 : Constant  Value=0.3295
  Constant5 : Constant  Value=0.7273
  Constant6 : Constant  Value=0.7273
  Constant7 : Constant  Value=1.0
  Gain : Gain  Gain=0.009
  Gain1 : Gain  Gain=0.09637
  Gain2 : Gain  Gain=0.48563
  Gain3 : Gain  Gain=0.06768
  Gain4 : Gain  Gain=20
  MATLAB Function : MATLAB Function  TreatAsAtomicUnit=on
  MATLAB Function1 : MATLAB Function  TreatAsAtomicUnit=on
  MATLAB Function2 : MATLAB Function  TreatAsAtomicUnit=on
  MATLAB Function3 : MATLAB Function  TreatAsAtomicUnit=on
  Out1 : Outport
  wires:
  Gain4/1 -> Out1/1
  Add/1 -> Gain4/1
  MATLAB Function/1(y) -> Gain/1
  MATLAB Function1/1(y) -> Gain1/1
  MATLAB Function2/1(y) -> Gain2/1
  MATLAB Function3/1(y) -> Gain3/1
  Constant/1 -> MATLAB Function/2(a)
  Constant1/1 -> MATLAB Function/3(b)
  Constant2/1 -> MATLAB Function1/2(a)
  Constant3/1 -> MATLAB Function1/3(b)
  Constant4/1 -> MATLAB Function2/2(a)
  Constant5/1 -> MATLAB Function2/3(b)
  Constant6/1 -> MATLAB Function3/2(a)
  Constant7/1 -> MATLAB Function3/3(b)
  Gain/1 -> Add/1
  Gain1/1 -> Add/2
  Gain2/1 -> Add/3
  Gain3/1 -> Add/4
  u1/1 -> MATLAB Function3/1(u), MATLAB Function2/1(u), MATLAB Function/1(u), MATLAB Function1/1(u)

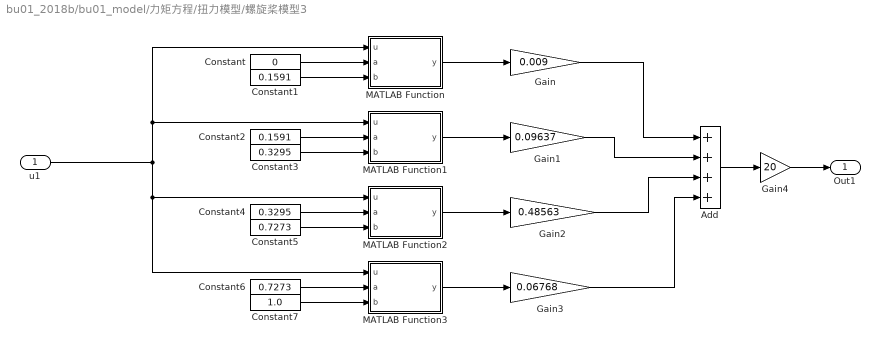
== system bu01_2018b/bu01_model/力矩方程/扭力模型/螺旋桨模型3 ==
  u1 : Inport
  Add : Sum  Inputs=4
  Constant : Constant  Value=0
  Constant1 : Constant  Value=0.1591
  Constant2 : Constant  Value=0.1591
  Constant3 : Constant  Value=0.3295
  Constant4 : Constant  Value=0.3295
  Constant5 : Constant  Value=0.7273
  Constant6 : Constant  Value=0.7273
  Constant7 : Constant  Value=1.0
  Gain : Gain  Gain=0.009
  Gain1 : Gain  Gain=0.09637
  Gain2 : Gain  Gain=0.48563
  Gain3 : Gain  Gain=0.06768
  Gain4 : Gain  Gain=20
  MATLAB Function : MATLAB Function  TreatAsAtomicUnit=on
  MATLAB Function1 : MATLAB Function  TreatAsAtomicUnit=on
  MATLAB Function2 : MATLAB Function  TreatAsAtomicUnit=on
  MATLAB Function3 : MATLAB Function  TreatAsAtomicUnit=on
  Out1 : Outport
  wires:
  u1/1 -> MATLAB Function1/1(u), MATLAB Function/1(u), MATLAB Function2/1(u), MATLAB Function3/1(u)
  Gain3/1 -> Add/4
  Gain2/1 -> Add/3
  Gain1/1 -> Add/2
  Gain/1 -> Add/1
  Constant7/1 -> MATLAB Function3/3(b)
  Constant6/1 -> MATLAB Function3/2(a)
  Constant5/1 -> MATLAB Function2/3(b)
  Constant4/1 -> MATLAB Function2/2(a)
  Constant3/1 -> MATLAB Function1/3(b)
  Constant2/1 -> MATLAB Function1/2(a)
  Constant1/1 -> MATLAB Function/3(b)
  Constant/1 -> MATLAB Function/2(a)
  MATLAB Function3/1(y) -> Gain3/1
  MATLAB Function2/1(y) -> Gain2/1
  MATLAB Function1/1(y) -> Gain1/1
  MATLAB Function/1(y) -> Gain/1
  Add/1 -> Gain4/1
  Gain4/1 -> Out1/1

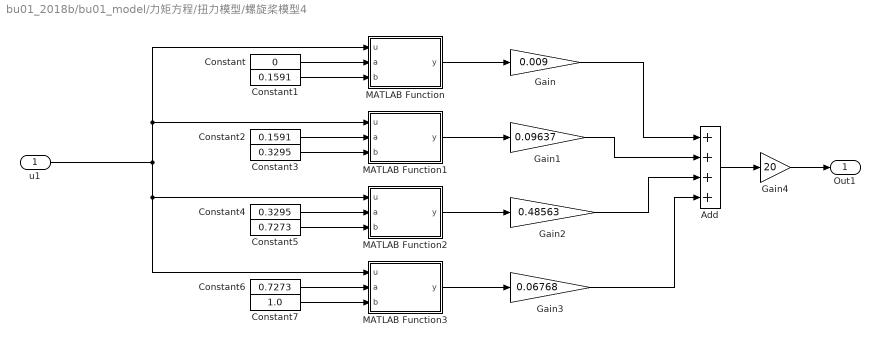
== system bu01_2018b/bu01_model/力矩方程/扭力模型/螺旋桨模型4 ==
  u1 : Inport
  Add : Sum  Inputs=4
  Constant : Constant  Value=0
  Constant1 : Constant  Value=0.1591
  Constant2 : Constant  Value=0.1591
  Constant3 : Constant  Value=0.3295
  Constant4 : Constant  Value=0.3295
  Constant5 : Constant  Value=0.7273
  Constant6 : Constant  Value=0.7273
  Constant7 : Constant  Value=1.0
  Gain : Gain  Gain=0.009
  Gain1 : Gain  Gain=0.09637
  Gain2 : Gain  Gain=0.48563
  Gain3 : Gain  Gain=0.06768
  Gain4 : Gain  Gain=20
  MATLAB Function : MATLAB Function  TreatAsAtomicUnit=on
  MATLAB Function1 : MATLAB Function  TreatAsAtomicUnit=on
  MATLAB Function2 : MATLAB Function  TreatAsAtomicUnit=on
  MATLAB Function3 : MATLAB Function  TreatAsAtomicUnit=on
  Out1 : Outport
  wires:
  Gain4/1 -> Out1/1
  Add/1 -> Gain4/1
  MATLAB Function/1(y) -> Gain/1
  MATLAB Function1/1(y) -> Gain1/1
  MATLAB Function2/1(y) -> Gain2/1
  MATLAB Function3/1(y) -> Gain3/1
  Constant/1 -> MATLAB Function/2(a)
  Constant1/1 -> MATLAB Function/3(b)
  Constant2/1 -> MATLAB Function1/2(a)
  Constant3/1 -> MATLAB Function1/3(b)
  Constant4/1 -> MATLAB Function2/2(a)
  Constant5/1 -> MATLAB Function2/3(b)
  Constant6/1 -> MATLAB Function3/2(a)
  Constant7/1 -> MATLAB Function3/3(b)
  Gain/1 -> Add/1
  Gain1/1 -> Add/2
  Gain2/1 -> Add/3
  Gain3/1 -> Add/4
  u1/1 -> MATLAB Function3/1(u), MATLAB Function2/1(u), MATLAB Function/1(u), MATLAB Function1/1(u)

== system bu01_2018b/bu01_model/力矩方程/推力模型/涵道模型模型1 ==
  u1 : Inport
  Add : Sum
  Constant : Constant  Value=0
  Constant1 : Constant  Value=0.1023
  Constant2 : Constant  Value=0.1023
  Constant3 : Constant
  Gain : Gain  Gain=21
  Gain1 : Gain  Gain=2.4013e+03
  MATLAB Function : MATLAB Function  TreatAsAtomicUnit=on
  MATLAB Function1 : MATLAB Function  TreatAsAtomicUnit=on
  Out1 : Outport
  wires:
  MATLAB Function1/1(y) -> Gain1/1
  Constant2/1 -> MATLAB Function1/2(a)
  Constant3/1 -> MATLAB Function1/3(b)
  Constant1/1 -> MATLAB Function/3(b)
  Gain1/1 -> Add/2
  Constant/1 -> MATLAB Function/2(a)
  u1/1 -> MATLAB Function1/1(u), MATLAB Function/1(u)
  Gain/1 -> Add/1
  MATLAB Function/1(y) -> Gain/1
  Add/1 -> Out1/1

== system bu01_2018b/bu01_model/力矩方程/推力模型/涵道模型模型2 ==
  u1 : Inport
  Add : Sum
  Constant : Constant  Value=0
  Constant1 : Constant  Value=0.1023
  Constant2 : Constant  Value=0.1023
  Constant3 : Constant
  Gain : Gain  Gain=21
  Gain1 : Gain  Gain=2.4013e+03
  MATLAB Function : MATLAB Function  TreatAsAtomicUnit=on
  MATLAB Function1 : MATLAB Function  TreatAsAtomicUnit=on
  Out1 : Outport
  wires:
  Add/1 -> Out1/1
  MATLAB Function/1(y) -> Gain/1
  Gain/1 -> Add/1
  u1/1 -> MATLAB Function/1(u), MATLAB Function1/1(u)
  Constant/1 -> MATLAB Function/2(a)
  Gain1/1 -> Add/2
  Constant1/1 -> MATLAB Function/3(b)
  Constant3/1 -> MATLAB Function1/3(b)
  Constant2/1 -> MATLAB Function1/2(a)
  MATLAB Function1/1(y) -> Gain1/1

== system bu01_2018b/bu01_model/力矩方程/推力模型/涵道模型模型3 ==
  u1 : Inport
  Add : Sum
  Constant : Constant  Value=0
  Constant1 : Constant  Value=0.1023
  Constant2 : Constant  Value=0.1023
  Constant3 : Constant
  Gain : Gain  Gain=21
  Gain1 : Gain  Gain=2.4013e+03
  MATLAB Function : MATLAB Function  TreatAsAtomicUnit=on
  MATLAB Function1 : MATLAB Function  TreatAsAtomicUnit=on
  Out1 : Outport
  wires:
  MATLAB Function1/1(y) -> Gain1/1
  Constant2/1 -> MATLAB Function1/2(a)
  Constant3/1 -> MATLAB Function1/3(b)
  Constant1/1 -> MATLAB Function/3(b)
  Gain1/1 -> Add/2
  Constant/1 -> MATLAB Function/2(a)
  u1/1 -> MATLAB Function1/1(u), MATLAB Function/1(u)
  Gain/1 -> Add/1
  MATLAB Function/1(y) -> Gain/1
  Add/1 -> Out1/1

== system bu01_2018b/bu01_model/力矩方程/推力模型/涵道模型模型4 ==
  u1 : Inport
  Add : Sum
  Constant : Constant  Value=0
  Constant1 : Constant  Value=0.1023
  Constant2 : Constant  Value=0.1023
  Constant3 : Constant
  Gain : Gain  Gain=21
  Gain1 : Gain  Gain=2.4013e+03
  MATLAB Function : MATLAB Function  TreatAsAtomicUnit=on
  MATLAB Function1 : MATLAB Function  TreatAsAtomicUnit=on
  Out1 : Outport
  wires:
  Add/1 -> Out1/1
  MATLAB Function/1(y) -> Gain/1
  Gain/1 -> Add/1
  u1/1 -> MATLAB Function/1(u), MATLAB Function1/1(u)
  Constant/1 -> MATLAB Function/2(a)
  Gain1/1 -> Add/2
  Constant1/1 -> MATLAB Function/3(b)
  Constant3/1 -> MATLAB Function1/3(b)
  Constant2/1 -> MATLAB Function1/2(a)
  MATLAB Function1/1(y) -> Gain1/1

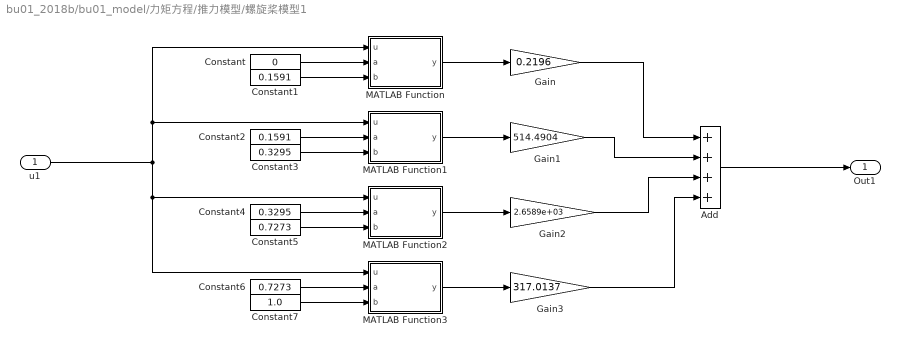
== system bu01_2018b/bu01_model/力矩方程/推力模型/螺旋桨模型1 ==
  u1 : Inport
  Add : Sum  Inputs=4
  Constant : Constant  Value=0
  Constant1 : Constant  Value=0.1591
  Constant2 : Constant  Value=0.1591
  Constant3 : Constant  Value=0.3295
  Constant4 : Constant  Value=0.3295
  Constant5 : Constant  Value=0.7273
  Constant6 : Constant  Value=0.7273
  Constant7 : Constant  Value=1.0
  Gain : Gain  Gain=0.2196
  Gain1 : Gain  Gain=514.4904
  Gain2 : Gain  Gain=2.6589e+03
  Gain3 : Gain  Gain=317.0137
  MATLAB Function : MATLAB Function  TreatAsAtomicUnit=on
  MATLAB Function1 : MATLAB Function  TreatAsAtomicUnit=on
  MATLAB Function2 : MATLAB Function  TreatAsAtomicUnit=on
  MATLAB Function3 : MATLAB Function  TreatAsAtomicUnit=on
  Out1 : Outport
  wires:
  Add/1 -> Out1/1
  u1/1 -> MATLAB Function1/1(u), MATLAB Function/1(u), MATLAB Function2/1(u), MATLAB Function3/1(u)
  Gain3/1 -> Add/4
  Gain2/1 -> Add/3
  Gain1/1 -> Add/2
  Gain/1 -> Add/1
  Constant7/1 -> MATLAB Function3/3(b)
  Constant6/1 -> MATLAB Function3/2(a)
  Constant5/1 -> MATLAB Function2/3(b)
  Constant4/1 -> MATLAB Function2/2(a)
  Constant3/1 -> MATLAB Function1/3(b)
  Constant2/1 -> MATLAB Function1/2(a)
  Constant1/1 -> MATLAB Function/3(b)
  Constant/1 -> MATLAB Function/2(a)
  MATLAB Function3/1(y) -> Gain3/1
  MATLAB Function2/1(y) -> Gain2/1
  MATLAB Function1/1(y) -> Gain1/1
  MATLAB Function/1(y) -> Gain/1

== system bu01_2018b/bu01_model/力矩方程/推力模型/螺旋桨模型2 ==
  u1 : Inport
  Add : Sum  Inputs=4
  Constant : Constant  Value=0
  Constant1 : Constant  Value=0.1591
  Constant2 : Constant  Value=0.1591
  Constant3 : Constant  Value=0.3295
  Constant4 : Constant  Value=0.3295
  Constant5 : Constant  Value=0.7273
  Constant6 : Constant  Value=0.7273
  Constant7 : Constant  Value=1.0
  Gain : Gain  Gain=0.2196
  Gain1 : Gain  Gain=514.4904
  Gain2 : Gain  Gain=2.6589e+03
  Gain3 : Gain  Gain=317.0137
  MATLAB Function : MATLAB Function  TreatAsAtomicUnit=on
  MATLAB Function1 : MATLAB Function  TreatAsAtomicUnit=on
  MATLAB Function2 : MATLAB Function  TreatAsAtomicUnit=on
  MATLAB Function3 : MATLAB Function  TreatAsAtomicUnit=on
  Out1 : Outport
  wires:
  MATLAB Function/1(y) -> Gain/1
  MATLAB Function1/1(y) -> Gain1/1
  MATLAB Function2/1(y) -> Gain2/1
  MATLAB Function3/1(y) -> Gain3/1
  Constant/1 -> MATLAB Function/2(a)
  Constant1/1 -> MATLAB Function/3(b)
  Constant2/1 -> MATLAB Function1/2(a)
  Constant3/1 -> MATLAB Function1/3(b)
  Constant4/1 -> MATLAB Function2/2(a)
  Constant5/1 -> MATLAB Function2/3(b)
  Constant6/1 -> MATLAB Function3/2(a)
  Constant7/1 -> MATLAB Function3/3(b)
  Gain/1 -> Add/1
  Gain1/1 -> Add/2
  Gain2/1 -> Add/3
  Gain3/1 -> Add/4
  u1/1 -> MATLAB Function3/1(u), MATLAB Function2/1(u), MATLAB Function/1(u), MATLAB Function1/1(u)
  Add/1 -> Out1/1

== system bu01_2018b/bu01_model/力矩方程/推力模型/螺旋桨模型3 ==
  u1 : Inport
  Add : Sum  Inputs=4
  Constant : Constant  Value=0
  Constant1 : Constant  Value=0.1591
  Constant2 : Constant  Value=0.1591
  Constant3 : Constant  Value=0.3295
  Constant4 : Constant  Value=0.3295
  Constant5 : Constant  Value=0.7273
  Constant6 : Constant  Value=0.7273
  Constant7 : Constant  Value=1.0
  Gain : Gain  Gain=0.2196
  Gain1 : Gain  Gain=514.4904
  Gain2 : Gain  Gain=2.6589e+03
  Gain3 : Gain  Gain=317.0137
  MATLAB Function : MATLAB Function  TreatAsAtomicUnit=on
  MATLAB Function1 : MATLAB Function  TreatAsAtomicUnit=on
  MATLAB Function2 : MATLAB Function  TreatAsAtomicUnit=on
  MATLAB Function3 : MATLAB Function  TreatAsAtomicUnit=on
  Out1 : Outport
  wires:
  Add/1 -> Out1/1
  u1/1 -> MATLAB Function1/1(u), MATLAB Function/1(u), MATLAB Function2/1(u), MATLAB Function3/1(u)
  Gain3/1 -> Add/4
  Gain2/1 -> Add/3
  Gain1/1 -> Add/2
  Gain/1 -> Add/1
  Constant7/1 -> MATLAB Function3/3(b)
  Constant6/1 -> MATLAB Function3/2(a)
  Constant5/1 -> MATLAB Function2/3(b)
  Constant4/1 -> MATLAB Function2/2(a)
  Constant3/1 -> MATLAB Function1/3(b)
  Constant2/1 -> MATLAB Function1/2(a)
  Constant1/1 -> MATLAB Function/3(b)
  Constant/1 -> MATLAB Function/2(a)
  MATLAB Function3/1(y) -> Gain3/1
  MATLAB Function2/1(y) -> Gain2/1
  MATLAB Function1/1(y) -> Gain1/1
  MATLAB Function/1(y) -> Gain/1

== system bu01_2018b/bu01_model/力矩方程/推力模型/螺旋桨模型4 ==
  u1 : Inport
  Add : Sum  Inputs=4
  Constant : Constant  Value=0
  Constant1 : Constant  Value=0.1591
  Constant2 : Constant  Value=0.1591
  Constant3 : Constant  Value=0.3295
  Constant4 : Constant  Value=0.3295
  Constant5 : Constant  Value=0.7273
  Constant6 : Constant  Value=0.7273
  Constant7 : Constant  Value=1.0
  Gain : Gain  Gain=0.2196
  Gain1 : Gain  Gain=514.4904
  Gain2 : Gain  Gain=2.6589e+03
  Gain3 : Gain  Gain=317.0137
  MATLAB Function : MATLAB Function  TreatAsAtomicUnit=on
  MATLAB Function1 : MATLAB Function  TreatAsAtomicUnit=on
  MATLAB Function2 : MATLAB Function  TreatAsAtomicUnit=on
  MATLAB Function3 : MATLAB Function  TreatAsAtomicUnit=on
  Out1 : Outport
  wires:
  MATLAB Function/1(y) -> Gain/1
  MATLAB Function1/1(y) -> Gain1/1
  MATLAB Function2/1(y) -> Gain2/1
  MATLAB Function3/1(y) -> Gain3/1
  Constant/1 -> MATLAB Function/2(a)
  Constant1/1 -> MATLAB Function/3(b)
  Constant2/1 -> MATLAB Function1/2(a)
  Constant3/1 -> MATLAB Function1/3(b)
  Constant4/1 -> MATLAB Function2/2(a)
  Constant5/1 -> MATLAB Function2/3(b)
  Constant6/1 -> MATLAB Function3/2(a)
  Constant7/1 -> MATLAB Function3/3(b)
  Gain/1 -> Add/1
  Gain1/1 -> Add/2
  Gain2/1 -> Add/3
  Gain3/1 -> Add/4
  u1/1 -> MATLAB Function3/1(u), MATLAB Function2/1(u), MATLAB Function/1(u), MATLAB Function1/1(u)
  Add/1 -> Out1/1

== system bu01_2018b/bu01_model/推力方程/动力模型/涵道模型模型1 ==
  u1 : Inport
  Add : Sum
  Constant : Constant  Value=0
  Constant1 : Constant  Value=0.1023
  Constant2 : Constant  Value=0.1023
  Constant3 : Constant
  Gain : Gain  Gain=21
  Gain1 : Gain  Gain=2.4013e+03
  MATLAB Function : MATLAB Function  TreatAsAtomicUnit=on
  MATLAB Function1 : MATLAB Function  TreatAsAtomicUnit=on
  Out1 : Outport
  wires:
  MATLAB Function1/1(y) -> Gain1/1
  Constant2/1 -> MATLAB Function1/2(a)
  Constant3/1 -> MATLAB Function1/3(b)
  Constant1/1 -> MATLAB Function/3(b)
  Gain1/1 -> Add/2
  Constant/1 -> MATLAB Function/2(a)
  u1/1 -> MATLAB Function1/1(u), MATLAB Function/1(u)
  Gain/1 -> Add/1
  MATLAB Function/1(y) -> Gain/1
  Add/1 -> Out1/1

== system bu01_2018b/bu01_model/推力方程/动力模型/涵道模型模型2 ==
  u1 : Inport
  Add : Sum
  Constant : Constant  Value=0
  Constant1 : Constant  Value=0.1023
  Constant2 : Constant  Value=0.1023
  Constant3 : Constant
  Gain : Gain  Gain=21
  Gain1 : Gain  Gain=2.4013e+03
  MATLAB Function : MATLAB Function  TreatAsAtomicUnit=on
  MATLAB Function1 : MATLAB Function  TreatAsAtomicUnit=on
  Out1 : Outport
  wires:
  Add/1 -> Out1/1
  MATLAB Function/1(y) -> Gain/1
  Gain/1 -> Add/1
  u1/1 -> MATLAB Function/1(u), MATLAB Function1/1(u)
  Constant/1 -> MATLAB Function/2(a)
  Gain1/1 -> Add/2
  Constant1/1 -> MATLAB Function/3(b)
  Constant3/1 -> MATLAB Function1/3(b)
  Constant2/1 -> MATLAB Function1/2(a)
  MATLAB Function1/1(y) -> Gain1/1

== system bu01_2018b/bu01_model/推力方程/动力模型/涵道模型模型3 ==
  u1 : Inport
  Add : Sum
  Constant : Constant  Value=0
  Constant1 : Constant  Value=0.1023
  Constant2 : Constant  Value=0.1023
  Constant3 : Constant
  Gain : Gain  Gain=21
  Gain1 : Gain  Gain=2.4013e+03
  MATLAB Function : MATLAB Function  TreatAsAtomicUnit=on
  MATLAB Function1 : MATLAB Function  TreatAsAtomicUnit=on
  Out1 : Outport
  wires:
  MATLAB Function1/1(y) -> Gain1/1
  Constant2/1 -> MATLAB Function1/2(a)
  Constant3/1 -> MATLAB Function1/3(b)
  Constant1/1 -> MATLAB Function/3(b)
  Gain1/1 -> Add/2
  Constant/1 -> MATLAB Function/2(a)
  u1/1 -> MATLAB Function1/1(u), MATLAB Function/1(u)
  Gain/1 -> Add/1
  MATLAB Function/1(y) -> Gain/1
  Add/1 -> Out1/1

== system bu01_2018b/bu01_model/推力方程/动力模型/涵道模型模型4 ==
  u1 : Inport
  Add : Sum
  Constant : Constant  Value=0
  Constant1 : Constant  Value=0.1023
  Constant2 : Constant  Value=0.1023
  Constant3 : Constant
  Gain : Gain  Gain=21
  Gain1 : Gain  Gain=2.4013e+03
  MATLAB Function : MATLAB Function  TreatAsAtomicUnit=on
  MATLAB Function1 : MATLAB Function  TreatAsAtomicUnit=on
  Out1 : Outport
  wires:
  Add/1 -> Out1/1
  MATLAB Function/1(y) -> Gain/1
  Gain/1 -> Add/1
  u1/1 -> MATLAB Function/1(u), MATLAB Function1/1(u)
  Constant/1 -> MATLAB Function/2(a)
  Gain1/1 -> Add/2
  Constant1/1 -> MATLAB Function/3(b)
  Constant3/1 -> MATLAB Function1/3(b)
  Constant2/1 -> MATLAB Function1/2(a)
  MATLAB Function1/1(y) -> Gain1/1
